simulink subsystem "torqueCommand"  (R2022b)
settings: Solver=VariableStepAuto  StartTime=0.0  StopTime=10.0  RelTol=1e-3
libraries: Raptor_lib x1, torqueCommand_lib x1
settings Model: Creator=serga  LastModifiedBy=serga

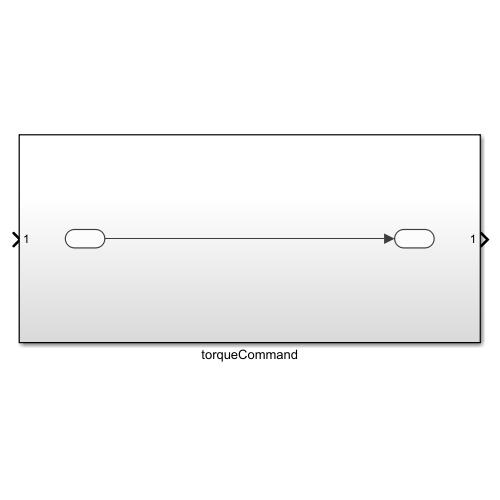
[thumbnail: Simulink's stored preview of the top-level diagram]
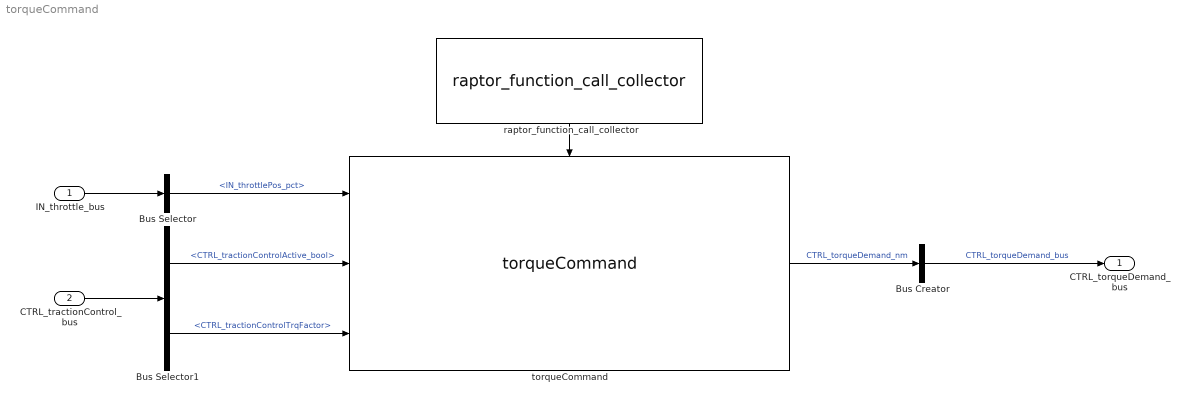
== system torqueCommand ==
  IN_throttle_bus : Inport
  CTRL_tractionControl_bus : Inport  Port=2
  Bus Creator : BusCreator  Inputs=1
  Bus Selector : BusSelector  OutputSignals=IN_throttlePos_pct
  Bus Selector1 : BusSelector  OutputSignals=CTRL_tractionControlActive_bool,CTRL_tractionControlTrqFactor
  raptor_function_call_collector : Raptor_lib/Triggers/raptor_function_call_collector  count=5
      settings: SourceProductName=Raptor
  torqueCommand : torqueCommand_lib/torqueCommand  SystemSampleTime=-1  VariantActivationTime=update diagram  Latency=0  AutoFrameSizeCalculation=off
  CTRL_torqueDemand_bus : Outport
  wires:
  raptor_function_call_collector/1 -> torqueCommand/Trigger
  IN_throttle_bus/1 -> Bus Selector/1
  CTRL_tractionControl_bus/1 -> Bus Selector1/1
  Bus Selector1/1 -> torqueCommand/2  "<CTRL_tractionControlActive_bool>"
  Bus Selector1/2 -> torqueCommand/3  "<CTRL_tractionControlTrqFactor>"
  Bus Selector/1 -> torqueCommand/1  "<IN_throttlePos_pct>"
  torqueCommand/1 -> Bus Creator/1  "CTRL_torqueDemand_nm"
  Bus Creator/1 -> CTRL_torqueDemand_bus/1  "CTRL_torqueDemand_bus"
